simulink model "mypid"  (R2018b)
settings: Solver=VariableStepAuto  StartTime=0.0  StopTime=30.0  RelTol=1e-3
settings Model: Creator=student  LastModifiedBy=student

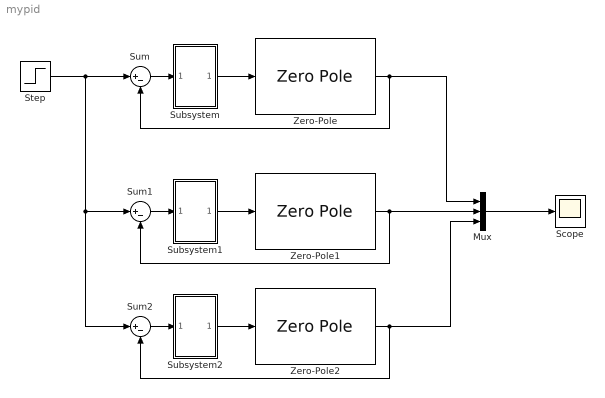
== system mypid ==
  Mux : Mux  Inputs=3
  Scope : Scope
  Step : Step  SampleTime=0
  Subsystem : Subsystem  mask{P=1, I=1, D=1}
  Subsystem1 : Subsystem  mask{P=1, I=1, D=1}
  Subsystem2 : Subsystem  mask{P=1, I=1, D=1}
  Sum : Sum  Inputs=|+-
  Sum1 : Sum  Inputs=|+-
  Sum2 : Sum  Inputs=|+-
  Zero-Pole : ZeroPole  Zeros=[]  Poles=[-1 -1 -1]
  Zero-Pole1 : ZeroPole  Zeros=[]  Poles=[-1 -1 -1]
  Zero-Pole2 : ZeroPole  Zeros=[]  Poles=[-1 -1 -1]
  wires:
  Sum/1 -> Subsystem/1(In1)
  Subsystem/1(Out1) -> Zero-Pole/1
  Sum1/1 -> Subsystem1/1(In1)
  Step/1 -> Sum1/1, Sum2/1, Sum/1
  Subsystem1/1(Out1) -> Zero-Pole1/1
  Sum2/1 -> Subsystem2/1(In1)
  Subsystem2/1(Out1) -> Zero-Pole2/1
  Mux/1 -> Scope/1
  Zero-Pole/1 -> Mux/1, Sum/2
  Zero-Pole1/1 -> Mux/2, Sum1/2
  Zero-Pole2/1 -> Mux/3, Sum2/2

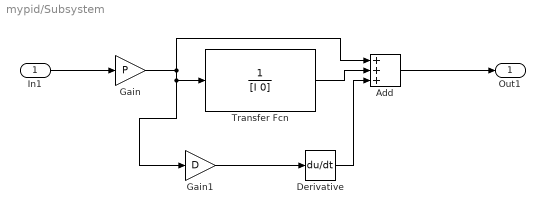
== system mypid/Subsystem ==
  In1 : Inport
  Add : Sum  Inputs=+++
  Derivative : Derivative
  Gain : Gain  Gain=P
  Gain1 : Gain  Gain=D
  Transfer Fcn : TransferFcn  Denominator=[I 0]
  Out1 : Outport
  wires:
  Gain1/1 -> Derivative/1
  Gain/1 -> Gain1/1, Transfer Fcn/1, Add/1
  Add/1 -> Out1/1
  In1/1 -> Gain/1
  Transfer Fcn/1 -> Add/2
  Derivative/1 -> Add/3

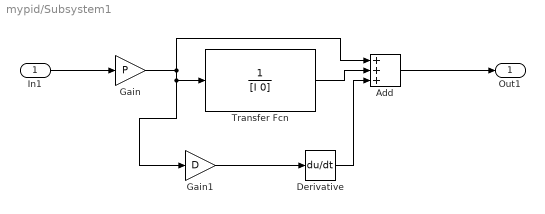
== system mypid/Subsystem1 ==
  In1 : Inport
  Add : Sum  Inputs=+++
  Derivative : Derivative
  Gain : Gain  Gain=P
  Gain1 : Gain  Gain=D
  Transfer Fcn : TransferFcn  Denominator=[I 0]
  Out1 : Outport
  wires:
  Gain1/1 -> Derivative/1
  Gain/1 -> Gain1/1, Transfer Fcn/1, Add/1
  Add/1 -> Out1/1
  In1/1 -> Gain/1
  Transfer Fcn/1 -> Add/2
  Derivative/1 -> Add/3

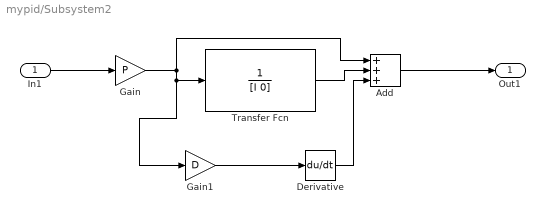
== system mypid/Subsystem2 ==
  In1 : Inport
  Add : Sum  Inputs=+++
  Derivative : Derivative
  Gain : Gain  Gain=P
  Gain1 : Gain  Gain=D
  Transfer Fcn : TransferFcn  Denominator=[I 0]
  Out1 : Outport
  wires:
  Gain1/1 -> Derivative/1
  Gain/1 -> Gain1/1, Transfer Fcn/1, Add/1
  Add/1 -> Out1/1
  In1/1 -> Gain/1
  Transfer Fcn/1 -> Add/2
  Derivative/1 -> Add/3
